simulink model "Model_simulink_pulse_Torque"  (R2017a)
settings: Solver=ode45  StartTime=0.0  StopTime=Tend  RelTol=1e-3
undefined symbols (not defined in the file): In, J, Kp, Kt, Kw, Lambda, m, Mn, psi, Rt, T, TR, Un, Uz0, V, wn, Y
settings Model: Creator=user  LastModifiedBy=a
settings DataIOCC: LimitDataPoints=on  SaveFormat=Array  SignalLoggingSaveFormat=ModelDataLogs
settings OptimizationCC: BlockReduction=off  BooleanDataType=off  ExpressionDepthLimit=2147483647  LifeSpan=inf
settings DebuggingCC: SaveWithParameterizedLinksMsg=none  UnderspecifiedInitializationDetection=Classic  MergeDetectMultiDrivingBlocksExec=none  SignalResolutionControl=TryResolveAllWithWarning  MultiTaskDSMMsg=warning  MultiTaskCondExecSysMsg=none  StateNameClashWarn=warning  SFUnexpectedBacktrackingDiag=warning  SFNoUnconditionalDefaultTransitionDiag=warning  SFExecutionAtInitializationDiag=none
settings HardwareCC: ProdBitPerPointer=32  ProdBitPerSizeT=32  ProdBitPerPtrDiffT=32  ProdLargestAtomicFloat=None  ProdIntDivRoundTo=Undefined  ProdEndianess=Unspecified  ProdWordSize=32  ProdHWDeviceType=32-bit Generic  TargetUnknown=on
settings ModelReferenceCC: PropagateSignalLabelsOutOfModel=off
settings GRTTargetCC: TargetLangStandard=C89/C90 (ANSI)  GeneratePreprocessorConditionals=Disable all
settings ConfigComp: CovMetricSettings=dw  CovHtmlReporting=on  CovSaveCumulativeToWorkspaceVar=on  CovSaveSingleToWorkspaceVar=on  CovExternalEMLEnable=off

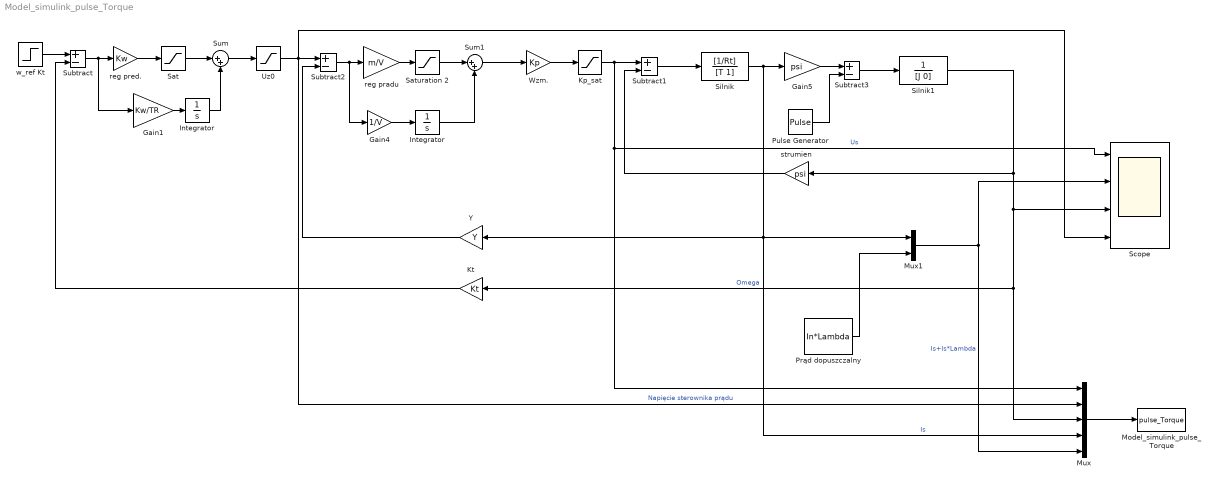
== system Model_simulink_pulse_Torque ==
  Gain1 : Gain  Gain=Kw/TR
  Gain4 : Gain  Gain=1/V
  Gain5 : Gain  Gain=psi
  Integrator : Integrator  LimitOutput=on  UpperSaturationLimit=10  LowerSaturationLimit=-10
  "Integrator " : Integrator  LimitOutput=on  UpperSaturationLimit=10  LowerSaturationLimit=-10
  Kp_sat : Saturate  UpperLimit=1.5*Un  LowerLimit=-1.5*Un
  Kt : Gain  Gain=Kt
  Model_simulink_pulse_Torque : ToWorkspace  VariableName=pulse_Torque  SaveFormat=Structure With Time  SampleTime=-1
  Mux : Mux  Inputs=5
  Mux1 : Mux  Inputs=2
  Prąd dopuszczalny : Constant  Value=In*Lambda
  Pulse Generator : DiscretePulseGenerator  PulseType=Time based  Amplitude=Mn  Period=3  PulseWidth=40  PhaseDelay=5
  Sat : Saturate  UpperLimit=10  LowerLimit=-10
  Saturation 2 : Saturate  UpperLimit=10  LowerLimit=-10
  Scope : Scope  NumInputPorts=4
  Silnik : TransferFcn  Numerator=[1/Rt]  Denominator=[T 1]
  Silnik1 : TransferFcn  Numerator=1  Denominator=[J 0]
  Subtract{,1..3} (4 alike) : Sum  Inputs=+-
  Sum : Sum  Inputs=|++
  Sum1 : Sum  Inputs=|++
  Uz0 : Saturate  UpperLimit=Uz0  LowerLimit=-Uz0
  Wzm. : Gain  Gain=Kp
  Y : Gain  Gain=Y
  reg pradu : Gain  Gain=m/V
  reg pred. : Gain  Gain=Kw
  strumien : Gain  Gain=psi
  w_ref Kt : Step  Time=0  After=wn*Kt  SampleTime=0
  wires:
  w_ref Kt/1 -> Subtract/1
  Subtract/1 -> Gain1/1, reg pred./1
  Gain1/1 -> Integrator/1
  reg pradu/1 -> Saturation 2/1
  Wzm./1 -> Kp_sat/1
  Gain4/1 -> "Integrator "/1
  Subtract1/1 -> Silnik/1
  Silnik/1 -> Mux/4, Y/1, Mux1/1, Gain5/1  "Is"
  Gain5/1 -> Subtract3/1
  Subtract3/1 -> Silnik1/1
  strumien/1 -> Subtract1/2
  Kp_sat/1 -> Mux/1, Scope/1, Subtract1/1  "Us"
  Y/1 -> Subtract2/2
  Mux1/1 -> Mux/5, Scope/2  "Is+Is*Lambda"
  Prąd dopuszczalny/1 -> Mux1/2
  Uz0/1 -> Mux/2, Scope/4, Subtract2/1  "Napięcie sterownika prądu"
  Silnik1/1 -> Mux/3, Kt/1, Scope/3, strumien/1  "Omega"
  Kt/1 -> Subtract/2
  reg pred./1 -> Sat/1
  Saturation 2/1 -> Sum1/1
  Sum1/1 -> Wzm./1
  "Integrator "/1 -> Sum1/2
  Subtract2/1 -> Gain4/1, reg pradu/1
  Sat/1 -> Sum/1
  Sum/1 -> Uz0/1
  Integrator/1 -> Sum/2
  Pulse Generator/1 -> Subtract3/2
  Mux/1 -> Model_simulink_pulse_Torque/1
